simulink model "BEV_Laengsdynamikmodell_v2"  (R2023b)
settings: configuration reference "SharedConfig" (kept outside this file)
undefined symbols (not defined in the file): acc_cycle_flag, Analyse, battery, battery_builder_rtmsupport, config_battery, config_gearbox, config_Inverter, config_motor, config_vehicle, GB, gcbh, gearbox_map, k_FW, ModuleAssembly1, ModuleType1, motormap, motormap2
libraries: powerlib x37, nesl_utility x18, GD_Batterymodel_NSGAII_1_lib x12, BatteryProtection x9, fl_lib x7, dspstat3 x4, simulink x3, eePmsmCurrentReferenceGen x2, spsControlledCurrentSourceLib x2, spsVoltageMeasurementLib x2, batt_lib x1, BatteryBalancing x1
(part 3 of 6)

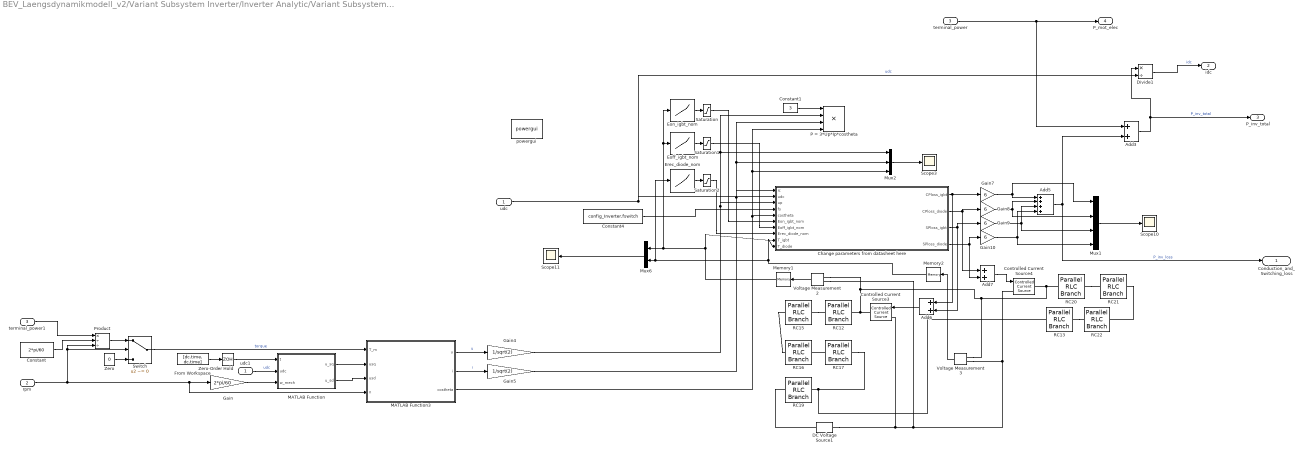
== system BEV_Laengsdynamikmodell_v2/Variant Subsystem Inverter/Inverter Analytic/Variant Subsystem/IM_Inverter_IGBT_Analytic ==
  udc : Inport
  rpm : Inport  Port=2
  terminal_power : Inport  Port=3
  Add3 : Sum
  Add5 : Sum  Inputs=++++
  Add6 : Sum
  Add7 : Sum
  Change parameters from datasheet here : MATLAB Function  TreatAsAtomicUnit=on
  Constant : Constant  Value=2*pi/60
  Constant1 : Constant  Value=3
  Constant4 : Constant  Value=config_Inverter.fswitch
  Controlled Current Source3 : powerlib/Electrical Sources/Controlled Current Source  Initialize=on  Source_Type=AC  Amplitude=0  Phase=0  Frequency=0  Measurements=None
  Controlled Current Source4 : powerlib/Electrical Sources/Controlled Current Source  Initialize=on  Source_Type=AC  Amplitude=0  Phase=0  Frequency=0  Measurements=None
  DC Voltage Source1 : powerlib/Electrical Sources/DC Voltage Source  Amplitude=25  Measurements=None
  Divide1 : Product  Inputs=*/
  Eoff_igbt_nom : Lookup_n-D  NumberOfTableDimensions=1  BreakpointsForDimension1=[25, 150, 175]  Table="[23.5*1e-3,  29*1e-3,  30*1e-3]"  InternalRulePriority=Speed  RndMeth=Simplest
  Eon_igbt_nom : Lookup_n-D  NumberOfTableDimensions=1  BreakpointsForDimension1=[25, 150, 175]  Table="[13.5*1e-3,  17.5*1e-3,  18*1e-3]"  InternalRulePriority=Speed  RndMeth=Simplest
  Erec_diode_nom : Lookup_n-D  NumberOfTableDimensions=1  BreakpointsForDimension1=[25, 150, 175]  Table="[7*1e-3,  13*1e-3,  15*1e-3]"  InternalRulePriority=Speed  RndMeth=Simplest
  From Workspace : FromWorkspace  VariableName=[dc.time, dc.time]
  Gain : Gain  Gain=2*pi/60
  Gain{7..10} (4 alike) : Gain  Gain=6
  Gain4 : Gain  Gain=1/sqrt(2)
  Gain5 : Gain  Gain=1/sqrt(2)
  MATLAB Function : MATLAB Function  TreatAsAtomicUnit=on
  MATLAB Function3 : MATLAB Function  TreatAsAtomicUnit=on
  Memory1 : Memory  InitialCondition=25  InheritSampleTime=on
  Memory2 : Memory  InitialCondition=25  InheritSampleTime=on
  Mux1 : Mux
  Mux2 : Mux  Inputs=3
  Mux6 : Mux  Inputs=2
  P = 3*Up*Ip*costheta : Product  Inputs=4
  Product : Product  Inputs=*//
  RC12 : powerlib/Elements/Parallel RLC Branch  LConnTagsString=a  RConnTagsString=__new0  BranchType=RC  Resistance=config_Inverter.R1igbt  Inductance=1e-3  SetiL0=off  InitialCurrent=0  Capacitance=config_Inverter.C1igbt  Setx0=off  InitialVoltage=0  Measurements=None
  RC13 : powerlib/Elements/Parallel RLC Branch  LConnTagsString=a  RConnTagsString=__new0  BranchType=RC  Resistance=config_Inverter.R4diode  Inductance=1e-3  SetiL0=off  InitialCurrent=0  Capacitance=config_Inverter.C4diode  Setx0=off  InitialVoltage=0  Measurements=None
  RC15 : powerlib/Elements/Parallel RLC Branch  LConnTagsString=a  RConnTagsString=__new0  BranchType=RC  Resistance=config_Inverter.R2igbt  Inductance=1e-3  SetiL0=off  InitialCurrent=0  Capacitance=config_Inverter.C2igbt  Setx0=off  InitialVoltage=0  Measurements=None
  RC16 : powerlib/Elements/Parallel RLC Branch  LConnTagsString=a  RConnTagsString=__new0  BranchType=RC  Resistance=config_Inverter.R3igbt  Inductance=1e-3  SetiL0=off  InitialCurrent=0  Capacitance=config_Inverter.C3igbt  Setx0=off  InitialVoltage=0  Measurements=None
  RC17 : powerlib/Elements/Parallel RLC Branch  LConnTagsString=a  RConnTagsString=__new0  BranchType=RC  Resistance=config_Inverter.R4igbt  Inductance=1e-3  SetiL0=off  InitialCurrent=0  Capacitance=config_Inverter.C4igbt  Setx0=off  InitialVoltage=0  Measurements=None
  RC19 : powerlib/Elements/Parallel RLC Branch  LConnTagsString=a  RConnTagsString=__new0  BranchType=R  Resistance=config_Inverter.R6igbt  Inductance=1e-3  SetiL0=off  InitialCurrent=0  Capacitance=175  Setx0=on  InitialVoltage=0  Measurements=None
  RC20 : powerlib/Elements/Parallel RLC Branch  LConnTagsString=a  RConnTagsString=__new0  BranchType=RC  Resistance=config_Inverter.R1diode  Inductance=1e-3  SetiL0=off  InitialCurrent=0  Capacitance=config_Inverter.C1diode  Setx0=off  InitialVoltage=0  Measurements=None
  RC21 : powerlib/Elements/Parallel RLC Branch  LConnTagsString=a  RConnTagsString=__new0  BranchType=RC  Resistance=config_Inverter.R2diode  Inductance=1e-3  SetiL0=off  InitialCurrent=0  Capacitance=config_Inverter.C2diode  Setx0=off  InitialVoltage=0  Measurements=None
  RC22 : powerlib/Elements/Parallel RLC Branch  LConnTagsString=a  RConnTagsString=__new0  BranchType=RC  Resistance=config_Inverter.R3diode  Inductance=1e-3  SetiL0=off  InitialCurrent=0  Capacitance=config_Inverter.C3diode  Setx0=off  InitialVoltage=0  Measurements=None
  Saturation : Saturate  UpperLimit=18*1e-3  LowerLimit=13.5*1e-3
  Saturation1 : Saturate  UpperLimit=30*1e-3  LowerLimit=23.5*1e-3
  Saturation2 : Saturate  UpperLimit=15*1e-3  LowerLimit=7*1e-3
  Scope10 : Scope
  Scope11 : Scope
  Scope3 : Scope
  Switch : Switch  Criteria=u2 ~= 0  SaturateOnIntegerOverflow=off  InputSameDT=off
  Voltage Measurement2 : powerlib/Measurements/Voltage Measurement  PhasorSimulation=off  OutputType=Complex  PSBequivalent=0
  Voltage Measurement3 : powerlib/Measurements/Voltage Measurement  PhasorSimulation=off  OutputType=Complex  PSBequivalent=0
  Zero : Constant  Value=0  OutDataTypeStr=Inherit: Inherit via back propagation
  Zero-Order Hold : ZeroOrderHold  SampleTime=-1
  powergui : powerlib/powergui  Priority=1  SimulationMode=Discrete  SampleTime=1  frequency=60  Iterations=50  frequencyindice=0  Pbase=100e6  ErrMax=1e-4  UnitsV=kV  UnitsW=MW  buscounter=0  FunctionMessages=on  echomessages=on  EnableUseOfTLC=off  CurrentSourceSwitches=off  DisableSnubberDevices=off  DisableRonSwitches=off  DisableVfSwitches=off  DisplayEquations=off  AutomaticDiscreteSolvers=off  SolverType=Backward Euler  Interpol=off  ExternalGateDelay=off  methode=off  Ts=100  x0status=blocks  SPID=off  SwTol=0  HookPort=off  NonlinearTolerance=1e-4  nMaxIteration=100  ContinueOnMaxIteration=off  RestoreLinks=warning  ResistiveCurrentMeasurement=off  Frange=[0:2:500]  Ylog=off  Xlog=on  ShowGrid=off  save=off  variable=ZData  structure=0  ZoomFFT=off  StartTime=0.0  cycles=1  DisplayStyle=1  fundamental=60  FreqAxis=off  MaxFrequency=1000  frequencyindicesteady=1  RmsSteady=1  display=off
  terminal_power1 : InportShadow  Port=3
  udc1 : InportShadow
  Conduction_and_Switching_loss : Outport
  idc : Outport  Port=2
  P_inv_total : Outport  Port=3
  P_mot_elec : Outport  Port=4
  wires:
  Eon_igbt_nom/1 -> Saturation/1
  Erec_diode_nom/1 -> Saturation2/1
  Eoff_igbt_nom/1 -> Saturation1/1
  Gain4/1 -> Change parameters from datasheet here/3(up), Mux2/1, P = 3*Up*Ip*costheta/2
  Saturation1/1 -> Change parameters from datasheet here/7(Eoff_igbt_nom)
  Switch/1 -> MATLAB Function3/1(T_m)  "torque"
  Divide1/1 -> idc/1  "idc"
  Voltage Measurement3/1 -> Memory2/1
  Change parameters from datasheet here/2(CPloss_diode) -> Add7/1, Gain8/1
  Add7/1 -> Controlled Current Source4/1
  Gain8/1 -> Add5/2, Mux1/2
  Change parameters from datasheet here/3(SPloss_igbt) -> Add6/2, Gain9/1
  Add3/1 -> Divide1/1, P_inv_total/1  "P_inv_total"
  Voltage Measurement2/1 -> Memory1/1
  Mux6/1 -> Scope11/1
  Saturation2/1 -> Change parameters from datasheet here/8(Erec_diode_nom)
  Saturation/1 -> Change parameters from datasheet here/6(Eon_igbt_nom)
  Change parameters from datasheet here/4(SPloss_diode) -> Add7/2, Gain10/1
  Gain9/1 -> Add5/3, Mux1/3
  Mux1/1 -> Scope10/1
  Gain7/1 -> Add5/1, Mux1/1
  Change parameters from datasheet here/1(CPloss_igbt) -> Gain7/1, Add6/1
  Constant4/1 -> Change parameters from datasheet here/4(fs)
  Memory1/1 -> Change parameters from datasheet here/9(T_igbt), Mux6/1, Eoff_igbt_nom/1, Eon_igbt_nom/1
  Memory2/1 -> Mux6/2, Erec_diode_nom/1, Change parameters from datasheet here/10(T_diode)
  Gain10/1 -> Mux1/4, Add5/4
  Constant1/1 -> P = 3*Up*Ip*costheta/1
  Add5/1 -> Add3/2, Conduction_and_Switching_loss/1  "P_inv_loss"
  Add6/1 -> Controlled Current Source3/1
  Mux2/1 -> Scope3/1
  udc/1 -> Divide1/2, Change parameters from datasheet here/2(udc)  "udc"
  MATLAB Function3/3(costheta) -> Mux2/3, P = 3*Up*Ip*costheta/4, Change parameters from datasheet here/5(costheta)
  Gain5/1 -> Change parameters from datasheet here/1(ic), Mux2/2, P = 3*Up*Ip*costheta/3
  MATLAB Function3/1(u) -> Gain4/1  "u"
  MATLAB Function3/2(i) -> Gain5/1  "i"
  MATLAB Function/1(u_sq) -> MATLAB Function3/2(usq)
  MATLAB Function/2(u_sd) -> MATLAB Function3/3(usd)
  Gain/1 -> MATLAB Function/3(w_mech)
  udc1/1 -> MATLAB Function/2(udc)  "udc"
  terminal_power/1 -> Add3/1, P_mot_elec/1
  Zero/1 -> Switch/3
  rpm/1 -> Switch/2, Product/3, MATLAB Function3/4(n), Gain/1
  Constant/1 -> Product/2
  Product/1 -> Switch/1
  terminal_power1/1 -> Product/1
  From Workspace/1 -> Zero-Order Hold/1
  Zero-Order Hold/1 -> MATLAB Function/1(t)
  connections:
  RC15/RConn1 -- RC12/LConn1
  RC17/LConn1 -- RC16/RConn1
  RC15/LConn1 -- RC16/LConn1
  RC20/LConn1 -- RC21/RConn1
  DC Voltage Source1/RConn1 -- RC19/LConn1
  RC13/LConn1 -- RC22/RConn1
  RC21/LConn1 -- RC22/LConn1
  RC17/RConn1 -- RC13/RConn1 -- RC19/RConn1
  Voltage Measurement2/LConn2 -- Voltage Measurement3/LConn2 -- Controlled Current Source4/LConn1 -- DC Voltage Source1/LConn1 -- Controlled Current Source3/LConn1
  RC12/RConn1 -- Controlled Current Source3/RConn1 -- Voltage Measurement2/LConn1 -- Voltage Measurement3/LConn1 -- RC20/RConn1 -- Controlled Current Source4/RConn1

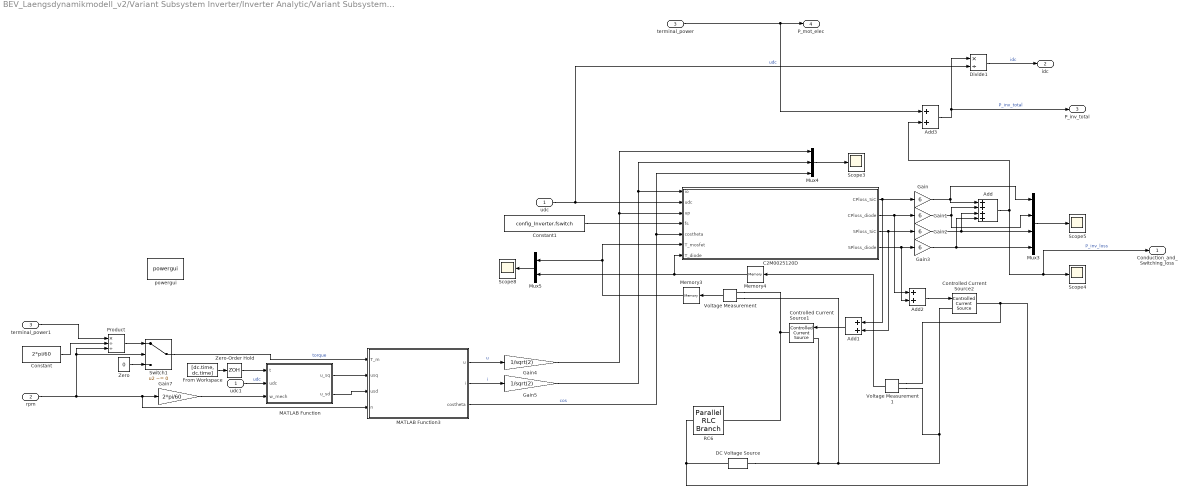
== system BEV_Laengsdynamikmodell_v2/Variant Subsystem Inverter/Inverter Analytic/Variant Subsystem/IM_Inverter_SiC-MOSFET_Analytic ==
  udc : Inport
  rpm : Inport  Port=2
  terminal_power : Inport  Port=3
  Add : Sum  Inputs=++++
  Add1 : Sum
  Add2 : Sum
  Add3 : Sum
  C2M0025120D : MATLAB Function  TreatAsAtomicUnit=on
  Constant : Constant  Value=2*pi/60
  Constant1 : Constant  Value=config_Inverter.fswitch
  Controlled Current Source1 : powerlib/Electrical Sources/Controlled Current Source  Initialize=on  Source_Type=AC  Amplitude=0  Phase=0  Frequency=0  Measurements=None
  Controlled Current Source2 : powerlib/Electrical Sources/Controlled Current Source  Initialize=on  Source_Type=AC  Amplitude=0  Phase=0  Frequency=0  Measurements=None
  DC Voltage Source : powerlib/Electrical Sources/DC Voltage Source  Amplitude=25  Measurements=None
  Divide1 : Product  Inputs=*/
  From Workspace : FromWorkspace  VariableName=[dc.time, dc.time]
  Gain{,1..3} (4 alike) : Gain  Gain=6
  Gain4 : Gain  Gain=1/sqrt(2)
  Gain5 : Gain  Gain=1/sqrt(2)
  Gain7 : Gain  Gain=2*pi/60
  MATLAB Function : MATLAB Function  TreatAsAtomicUnit=on
  MATLAB Function3 : MATLAB Function  TreatAsAtomicUnit=on
  Memory3 : Memory  InitialCondition=25  InheritSampleTime=on
  Memory4 : Memory  InitialCondition=25  InheritSampleTime=on
  Mux3 : Mux
  Mux4 : Mux  Inputs=3
  Mux5 : Mux  Inputs=2
  Product : Product  Inputs=*//
  RC6 : powerlib/Elements/Parallel RLC Branch  LConnTagsString=a  RConnTagsString=__new0  BranchType=R  Resistance=config_Inverter.Rmosfet  Inductance=1e-3  SetiL0=off  InitialCurrent=0  Capacitance=175  Setx0=on  InitialVoltage=0  Measurements=None
  Scope{3..5,8} (4 alike) : Scope
  Switch1 : Switch  Criteria=u2 ~= 0  SaturateOnIntegerOverflow=off  InputSameDT=off
  Voltage Measurement : powerlib/Measurements/Voltage Measurement  PhasorSimulation=off  OutputType=Complex  PSBequivalent=0
  Voltage Measurement1 : powerlib/Measurements/Voltage Measurement  PhasorSimulation=off  OutputType=Complex  PSBequivalent=0
  Zero : Constant  Value=0  OutDataTypeStr=Inherit: Inherit via back propagation
  Zero-Order Hold : ZeroOrderHold  SampleTime=-1
  powergui : powerlib/powergui  Priority=1  SimulationMode=Discrete  SampleTime=1  frequency=60  Iterations=50  frequencyindice=0  Pbase=100e6  ErrMax=1e-4  UnitsV=kV  UnitsW=MW  buscounter=0  FunctionMessages=on  echomessages=on  EnableUseOfTLC=off  CurrentSourceSwitches=off  DisableSnubberDevices=off  DisableRonSwitches=off  DisableVfSwitches=off  DisplayEquations=off  AutomaticDiscreteSolvers=off  SolverType=Backward Euler  Interpol=off  ExternalGateDelay=off  methode=off  Ts=100  x0status=blocks  SPID=off  SwTol=0  HookPort=off  NonlinearTolerance=1e-4  nMaxIteration=100  ContinueOnMaxIteration=off  RestoreLinks=warning  ResistiveCurrentMeasurement=off  Frange=[0:2:500]  Ylog=off  Xlog=on  ShowGrid=off  save=off  variable=ZData  structure=0  ZoomFFT=off  StartTime=0.0  cycles=1  DisplayStyle=1  fundamental=60  FreqAxis=off  MaxFrequency=1000  frequencyindicesteady=1  RmsSteady=1  display=off
  terminal_power1 : InportShadow  Port=3
  udc1 : InportShadow
  Conduction_and_Switching_loss : Outport
  idc : Outport  Port=2
  P_inv_total : Outport  Port=3
  P_mot_elec : Outport  Port=4
  wires:
  terminal_power/1 -> Add3/1, P_mot_elec/1
  Add3/1 -> Divide1/1, P_inv_total/1  "P_inv_total"
  Gain5/1 -> Mux4/2, C2M0025120D/1(io)
  Gain4/1 -> Mux4/1, C2M0025120D/3(up)
  udc/1 -> C2M0025120D/2(udc), Divide1/2  "udc"
  Divide1/1 -> idc/1  "idc"
  Add/1 -> Scope4/1, Conduction_and_Switching_loss/1, Add3/2  "P_inv_loss"
  MATLAB Function3/3(costheta) -> Mux4/3, C2M0025120D/5(costheta)  "cos"
  MATLAB Function3/2(i) -> Gain5/1  "i"
  Mux3/1 -> Scope5/1
  Mux4/1 -> Scope3/1
  Voltage Measurement/1 -> Memory3/1
  Mux5/1 -> Scope8/1
  C2M0025120D/2(CPloss_diode) -> Gain1/1, Add2/1
  Constant1/1 -> C2M0025120D/4(fs)
  C2M0025120D/3(SPloss_SiC) -> Gain2/1, Add1/2
  Voltage Measurement1/1 -> Memory4/1
  Add2/1 -> Controlled Current Source2/1
  Memory4/1 -> Mux5/2, C2M0025120D/7(T_diode)
  Add1/1 -> Controlled Current Source1/1
  Gain/1 -> Add/1, Mux3/1
  C2M0025120D/4(SPloss_diode) -> Gain3/1, Add2/2
  Gain1/1 -> Add/2, Mux3/2
  Gain2/1 -> Add/3, Mux3/3
  C2M0025120D/1(CPloss_SiC) -> Gain/1, Add1/1
  Memory3/1 -> C2M0025120D/6(T_mosfet), Mux5/1
  Gain3/1 -> Mux3/4, Add/4
  MATLAB Function/1(u_sq) -> MATLAB Function3/2(usq)
  MATLAB Function/2(u_sd) -> MATLAB Function3/3(usd)
  MATLAB Function3/1(u) -> Gain4/1  "u"
  terminal_power1/1 -> Product/1
  udc1/1 -> MATLAB Function/2(udc)  "udc"
  rpm/1 -> Switch1/2, Product/3, MATLAB Function3/4(n), Gain7/1
  Gain7/1 -> MATLAB Function/3(w_mech)
  Zero/1 -> Switch1/3
  Product/1 -> Switch1/1
  Constant/1 -> Product/2
  Switch1/1 -> MATLAB Function3/1(T_m)  "torque"
  From Workspace/1 -> Zero-Order Hold/1
  Zero-Order Hold/1 -> MATLAB Function/1(t)
  connections:
  RC6/RConn1 -- Controlled Current Source1/RConn1 -- Voltage Measurement/LConn1
  Controlled Current Source2/LConn1 -- Voltage Measurement/LConn2 -- Controlled Current Source1/LConn1 -- DC Voltage Source/LConn1 -- Voltage Measurement1/LConn2
  Voltage Measurement1/LConn1 -- Controlled Current Source2/RConn1 -- RC6/LConn1 -- DC Voltage Source/RConn1

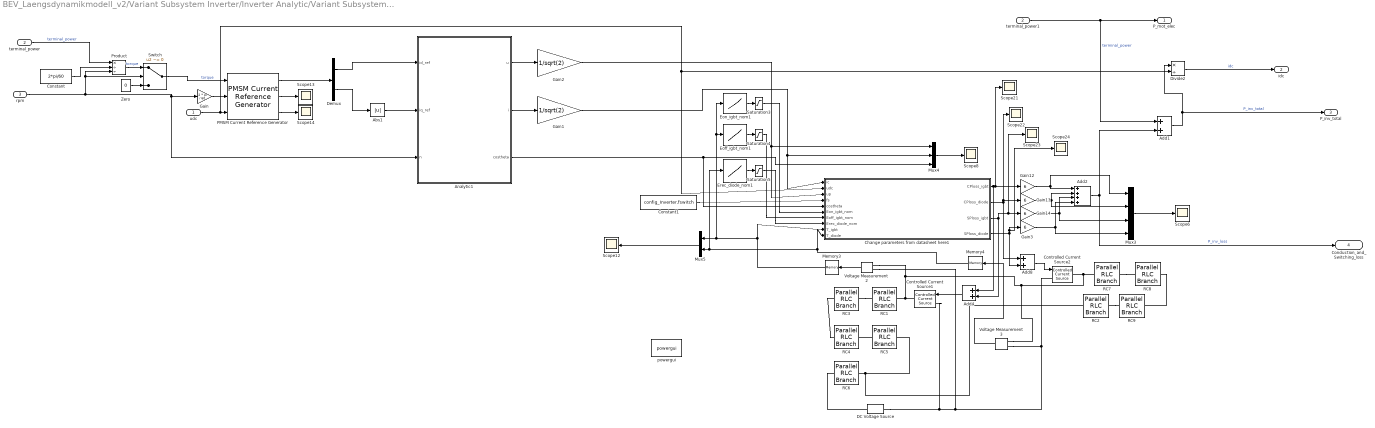
== system BEV_Laengsdynamikmodell_v2/Variant Subsystem Inverter/Inverter Analytic/Variant Subsystem/PMSM_Inverter_IBGT_Analytic ==
  udc : Inport
  terminal_power : Inport  Port=2
  rpm : Inport  Port=3
  Abs1 : Abs  SaturateOnIntegerOverflow=off
  Add1 : Sum
  Add2 : Sum  Inputs=++++
  Add4 : Sum
  Add8 : Sum
  Analytic1 : MATLAB Function  TreatAsAtomicUnit=on
  Change parameters from datasheet here1 : MATLAB Function  TreatAsAtomicUnit=on
  Constant : Constant  Value=2*pi/60
  Constant1 : Constant  Value=config_Inverter.fswitch
  Controlled Current Source1 : powerlib/Electrical Sources/Controlled Current Source  Initialize=on  Source_Type=AC  Amplitude=0  Phase=0  Frequency=0  Measurements=None
  Controlled Current Source2 : powerlib/Electrical Sources/Controlled Current Source  Initialize=on  Source_Type=AC  Amplitude=0  Phase=0  Frequency=0  Measurements=None
  DC Voltage Source : powerlib/Electrical Sources/DC Voltage Source  Amplitude=25  Measurements=None
  Demux : Demux  Outputs=2
  Divide2 : Product  Inputs=*/
  Eoff_igbt_nom1 : Lookup_n-D  NumberOfTableDimensions=1  BreakpointsForDimension1=[25, 150, 175]  Table="[23.5*1e-3,  29*1e-3,  30*1e-3]"  InternalRulePriority=Speed  RndMeth=Simplest
  Eon_igbt_nom1 : Lookup_n-D  NumberOfTableDimensions=1  BreakpointsForDimension1=[25, 150, 175]  Table="[13.5*1e-3,  17.5*1e-3,  18*1e-3]"  InternalRulePriority=Speed  RndMeth=Simplest
  Erec_diode_nom1 : Lookup_n-D  NumberOfTableDimensions=1  BreakpointsForDimension1=[25, 150, 175]  Table="[7*1e-3,  13*1e-3,  15*1e-3]"  InternalRulePriority=Speed  RndMeth=Simplest
  Gain : Gain  Gain=2 * pi / 60
  Gain1 : Gain  Gain=1/sqrt(2)
  Gain{3,12..14} (4 alike) : Gain  Gain=6
  Gain2 : Gain  Gain=1/sqrt(2)
  Memory3 : Memory  InitialCondition=25  InheritSampleTime=on
  Memory4 : Memory  InitialCondition=25  InheritSampleTime=on
  Mux3 : Mux
  Mux4 : Mux  Inputs=3
  Mux5 : Mux  Inputs=2
  PMSM Current Reference Generator : eePmsmCurrentReferenceGen/PMSM Current Reference Generator  Vnom=360  Pmax=150000  Tmax=350  Ts=-1  RefType=Automatically generated lookup-table  rpmVec=[0, 3000]  TqVec=[-100, 0, 100]  VdcVec=[300, 350]  PWMMode=SPWM: sinusoidal PWM  ModFactor=0.97  idMatrix=zeros(2,3,2)  iqMatrix=zeros(2,3,2)  p=6  psim=0.0347  Ld=0.0000436  Lq=0.0000975  Rs=0.0049  RefExpEnable=0
  Product : Product  Inputs=*//
  RC1 : powerlib/Elements/Parallel RLC Branch  LConnTagsString=a  RConnTagsString=__new0  BranchType=RC  Resistance=config_Inverter.R1igbt  Inductance=1e-3  SetiL0=off  InitialCurrent=0  Capacitance=config_Inverter.C1igbt  Setx0=off  InitialVoltage=0  Measurements=None
  RC2 : powerlib/Elements/Parallel RLC Branch  LConnTagsString=a  RConnTagsString=__new0  BranchType=RC  Resistance=config_Inverter.R4diode  Inductance=1e-3  SetiL0=off  InitialCurrent=0  Capacitance=config_Inverter.C4diode  Setx0=off  InitialVoltage=0  Measurements=None
  RC3 : powerlib/Elements/Parallel RLC Branch  LConnTagsString=a  RConnTagsString=__new0  BranchType=RC  Resistance=config_Inverter.R2igbt  Inductance=1e-3  SetiL0=off  InitialCurrent=0  Capacitance=config_Inverter.C2igbt  Setx0=off  InitialVoltage=0  Measurements=None
  RC4 : powerlib/Elements/Parallel RLC Branch  LConnTagsString=a  RConnTagsString=__new0  BranchType=RC  Resistance=config_Inverter.R3igbt  Inductance=1e-3  SetiL0=off  InitialCurrent=0  Capacitance=config_Inverter.C3igbt  Setx0=off  InitialVoltage=0  Measurements=None
  RC5 : powerlib/Elements/Parallel RLC Branch  LConnTagsString=a  RConnTagsString=__new0  BranchType=RC  Resistance=config_Inverter.R4igbt  Inductance=1e-3  SetiL0=off  InitialCurrent=0  Capacitance=config_Inverter.C4igbt  Setx0=off  InitialVoltage=0  Measurements=None
  RC6 : powerlib/Elements/Parallel RLC Branch  LConnTagsString=a  RConnTagsString=__new0  BranchType=R  Resistance=config_Inverter.R6igbt  Inductance=1e-3  SetiL0=off  InitialCurrent=0  Capacitance=175  Setx0=on  InitialVoltage=0  Measurements=None
  RC7 : powerlib/Elements/Parallel RLC Branch  LConnTagsString=a  RConnTagsString=__new0  BranchType=RC  Resistance=config_Inverter.R1diode  Inductance=1e-3  SetiL0=off  InitialCurrent=0  Capacitance=config_Inverter.C1diode  Setx0=off  InitialVoltage=0  Measurements=None
  RC8 : powerlib/Elements/Parallel RLC Branch  LConnTagsString=a  RConnTagsString=__new0  BranchType=RC  Resistance=config_Inverter.R2diode  Inductance=1e-3  SetiL0=off  InitialCurrent=0  Capacitance=config_Inverter.C2diode  Setx0=off  InitialVoltage=0  Measurements=None
  RC9 : powerlib/Elements/Parallel RLC Branch  LConnTagsString=a  RConnTagsString=__new0  BranchType=RC  Resistance=config_Inverter.R3diode  Inductance=1e-3  SetiL0=off  InitialCurrent=0  Capacitance=config_Inverter.C3diode  Setx0=off  InitialVoltage=0  Measurements=None
  Saturation3 : Saturate  UpperLimit=18*1e-3  LowerLimit=13.5*1e-3
  Saturation4 : Saturate  UpperLimit=30*1e-3  LowerLimit=23.5*1e-3
  Saturation5 : Saturate  UpperLimit=15*1e-3  LowerLimit=7*1e-3
  Scope{6,8,12..14,21..24} (9 alike) : Scope
  Switch : Switch  Criteria=u2 ~= 0  SaturateOnIntegerOverflow=off  InputSameDT=off
  Voltage Measurement2 : powerlib/Measurements/Voltage Measurement  PhasorSimulation=off  OutputType=Complex  PSBequivalent=0
  Voltage Measurement3 : powerlib/Measurements/Voltage Measurement  PhasorSimulation=off  OutputType=Complex  PSBequivalent=0
  Zero : Constant  Value=0  OutDataTypeStr=Inherit: Inherit via back propagation
  powergui : powerlib/powergui  Priority=1  SimulationMode=Discrete  SampleTime=1  frequency=60  Iterations=50  frequencyindice=0  Pbase=100e6  ErrMax=1e-4  UnitsV=kV  UnitsW=MW  buscounter=0  FunctionMessages=on  echomessages=on  EnableUseOfTLC=off  CurrentSourceSwitches=off  DisableSnubberDevices=off  DisableRonSwitches=off  DisableVfSwitches=off  DisplayEquations=off  AutomaticDiscreteSolvers=off  SolverType=Backward Euler  Interpol=off  ExternalGateDelay=off  methode=off  Ts=100  x0status=blocks  SPID=off  SwTol=0  HookPort=off  NonlinearTolerance=1e-4  nMaxIteration=100  ContinueOnMaxIteration=off  RestoreLinks=warning  ResistiveCurrentMeasurement=off  Frange=[0:2:500]  Ylog=off  Xlog=on  ShowGrid=off  save=off  variable=ZData  structure=0  ZoomFFT=off  StartTime=0.0  cycles=1  DisplayStyle=1  fundamental=60  FreqAxis=off  MaxFrequency=1000  frequencyindicesteady=1  RmsSteady=1  display=off
  terminal_power1 : InportShadow  Port=2
  P_mot_elec : Outport
  idc : Outport  Port=2
  P_inv_total : Outport  Port=3
  Conduction_and_Switching_loss : Outport  Port=4
  wires:
  PMSM Current Reference Generator/2 -> Scope13/1
  Eon_igbt_nom1/1 -> Saturation3/1
  Divide2/1 -> idc/1  "idc"
  Voltage Measurement2/1 -> Memory3/1
  Add8/1 -> Controlled Current Source2/1
  Change parameters from datasheet here1/3(SPloss_igbt) -> Scope23/1, Gain14/1, Add4/2
  Change parameters from datasheet here1/1(CPloss_igbt) -> Add4/1, Gain12/1, Scope21/1
  Gain2/1 -> Change parameters from datasheet here1/3(up), Mux4/1
  Add4/1 -> Controlled Current Source1/1
  Constant1/1 -> Change parameters from datasheet here1/4(fs)
  Eoff_igbt_nom1/1 -> Saturation4/1
  Saturation4/1 -> Change parameters from datasheet here1/7(Eoff_igbt_nom)
  PMSM Current Reference Generator/3 -> Scope14/1
  Demux/2 -> Abs1/1
  Change parameters from datasheet here1/2(CPloss_diode) -> Scope22/1, Gain13/1, Add8/1
  Voltage Measurement3/1 -> Memory4/1
  Memory3/1 -> Change parameters from datasheet here1/9(T_igbt), Eoff_igbt_nom1/1, Eon_igbt_nom1/1, Mux5/1
  Mux4/1 -> Scope8/1
  Mux5/1 -> Scope12/1
  Demux/1 -> Analytic1/1(id_ref)
  Memory4/1 -> Erec_diode_nom1/1, Mux5/2, Change parameters from datasheet here1/10(T_diode)
  Saturation5/1 -> Change parameters from datasheet here1/8(Erec_diode_nom)
  Add1/1 -> Divide2/1, P_inv_total/1  "P_inv_total"
  Analytic1/1(u) -> Gain2/1
  Erec_diode_nom1/1 -> Saturation5/1
  Mux3/1 -> Scope6/1
  Gain14/1 -> Mux3/3, Add2/3
  Gain/1 -> PMSM Current Reference Generator/2
  Add2/1 -> Conduction_and_Switching_loss/1, Add1/2  "P_inv_loss"
  Change parameters from datasheet here1/4(SPloss_diode) -> Scope24/1, Gain3/1, Add8/2
  Analytic1/2(i) -> Gain1/1
  PMSM Current Reference Generator/1 -> Demux/1
  Saturation3/1 -> Change parameters from datasheet here1/6(Eon_igbt_nom)
  Abs1/1 -> Analytic1/2(iq_ref)
  Gain13/1 -> Mux3/2, Add2/2
  rpm/1 -> Switch/2, Product/3, Analytic1/3(n), Gain/1
  terminal_power1/1 -> P_mot_elec/1, Add1/1  "terminal_power"
  Gain1/1 -> Change parameters from datasheet here1/1(ic), Mux4/2
  Gain12/1 -> Mux3/1, Add2/1
  udc/1 -> PMSM Current Reference Generator/3, Change parameters from datasheet here1/2(udc), Divide2/2
  Switch/1 -> PMSM Current Reference Generator/1  "torque"
  Gain3/1 -> Add2/4, Mux3/4
  Analytic1/3(costheta) -> Mux4/3, Change parameters from datasheet here1/5(costheta)
  terminal_power/1 -> Product/1  "terminal_power"
  Constant/1 -> Product/2
  Product/1 -> Switch/1  "torque"
  Zero/1 -> Switch/3
  connections:
  RC3/RConn1 -- RC1/LConn1
  RC7/LConn1 -- RC8/RConn1
  DC Voltage Source/RConn1 -- RC6/LConn1
  RC3/LConn1 -- RC4/LConn1
  RC5/LConn1 -- RC4/RConn1
  RC8/LConn1 -- RC9/LConn1
  Controlled Current Source1/LConn1 -- DC Voltage Source/LConn1 -- Voltage Measurement2/LConn1 -- Voltage Measurement3/LConn1 -- Controlled Current Source2/LConn1
  RC2/LConn1 -- RC9/RConn1
  RC5/RConn1 -- RC6/RConn1 -- RC2/RConn1
  Controlled Current Source2/RConn1 -- RC7/RConn1 -- Voltage Measurement3/LConn2 -- Voltage Measurement2/LConn2 -- Controlled Current Source1/RConn1 -- RC1/RConn1

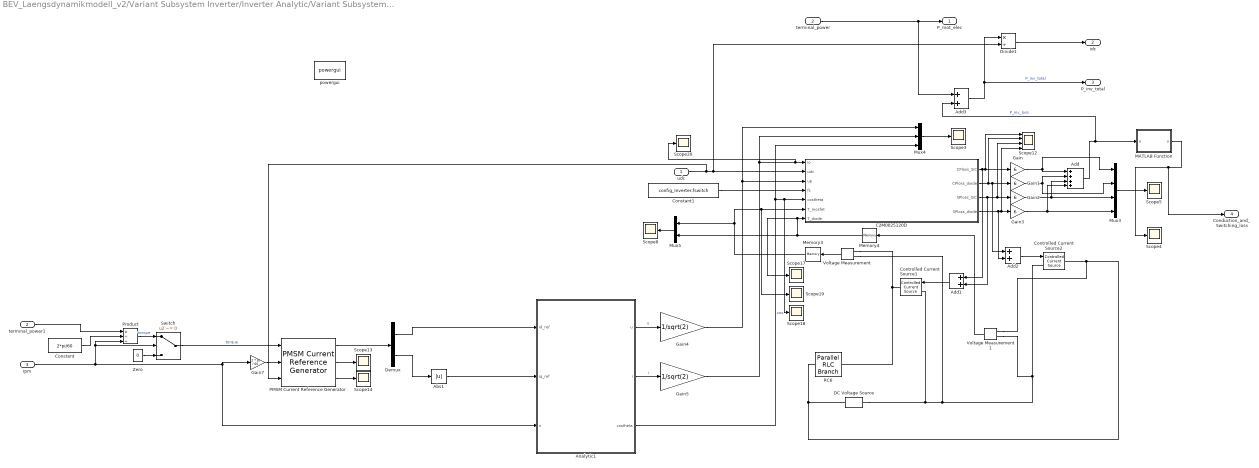
== system BEV_Laengsdynamikmodell_v2/Variant Subsystem Inverter/Inverter Analytic/Variant Subsystem/PMSM_Inverter_SiC-MOSFET_Analytic ==
  udc : Inport
  terminal_power : Inport  Port=2
  rpm : Inport  Port=3
  Abs1 : Abs  SaturateOnIntegerOverflow=off
  Add : Sum  Inputs=++++
  Add1 : Sum
  Add2 : Sum
  Add3 : Sum
  Analytic1 : MATLAB Function  TreatAsAtomicUnit=on
  C2M0025120D : MATLAB Function  TreatAsAtomicUnit=on
  Constant : Constant  Value=2*pi/60
  Constant1 : Constant  Value=config_Inverter.fswitch
  Controlled Current Source1 : spsControlledCurrentSourceLib/Controlled Current Source  Initialize=on  Source_Type=AC  Amplitude=0  Phase=0  Frequency=0  Measurements=None
  Controlled Current Source2 : spsControlledCurrentSourceLib/Controlled Current Source  Initialize=on  Source_Type=AC  Amplitude=0  Phase=0  Frequency=0  Measurements=None
  DC Voltage Source : spsDCVoltageSourceLib/DC Voltage Source  Amplitude=25  Measurements=None
  Demux : Demux  Outputs=2
  Divide1 : Product  Inputs=*/
  Gain{,1..3} (4 alike) : Gain  Gain=6
  Gain4 : Gain  Gain=1/sqrt(2)
  Gain5 : Gain  Gain=1/sqrt(2)
  Gain7 : Gain  Gain=2 * pi / 60
  MATLAB Function : MATLAB Function  TreatAsAtomicUnit=on
  Memory3 : Memory  InitialCondition=25  InheritSampleTime=on
  Memory4 : Memory  InitialCondition=25  InheritSampleTime=on
  Mux3 : Mux
  Mux4 : Mux  Inputs=3
  Mux5 : Mux  Inputs=2
  PMSM Current Reference Generator : eePmsmCurrentReferenceGen/PMSM Current Reference Generator  Vnom=360  Pmax=150000  Tmax=350  Ts=-1  RefType=Automatically generated lookup-table  rpmVec=[0, 3000]  TqVec=[-100, 0, 100]  VdcVec=[300, 350]  PWMMode=SPWM: sinusoidal PWM  ModFactor=0.97  idMatrix=zeros(2,3,2)  iqMatrix=zeros(2,3,2)  p=6  psim=0.0347  Ld=0.0000436  Lq=0.0000975  Rs=0.0049  RefExpEnable=0
  Product : Product  Inputs=*//
  RC6 : spsParallelRLCBranchLib/Parallel RLC Branch  LConnTagsString=a  RConnTagsString=__new0  BranchType=R  Resistance=config_Inverter.Rmosfet  Inductance=1e-3  SetiL0=off  InitialCurrent=0  Capacitance=175  Setx0=on  InitialVoltage=0  Measurements=None
  Scope12 : Scope  NumInputPorts=4
  Scope{3..5,8,13..14,17..20} (10 alike) : Scope
  Switch : Switch  Criteria=u2 ~= 0  SaturateOnIntegerOverflow=off  InputSameDT=off
  Voltage Measurement : spsVoltageMeasurementLib/Voltage Measurement  PhasorSimulation=off  OutputType=Complex  PSBequivalent=0
  Voltage Measurement1 : spsVoltageMeasurementLib/Voltage Measurement  PhasorSimulation=off  OutputType=Complex  PSBequivalent=0
  Zero : Constant  Value=0  OutDataTypeStr=Inherit: Inherit via back propagation
  powergui : spspowerguiLib/powergui  Priority=1  SimulationMode=Discrete  SampleTime=1  frequency=60  Iterations=50  frequencyindice=0  Pbase=100e6  ErrMax=1e-4  UnitsV=kV  UnitsW=MW  buscounter=0  FunctionMessages=on  echomessages=on  EnableUseOfTLC=off  CurrentSourceSwitches=off  DisableSnubberDevices=off  DisableRonSwitches=off  DisableVfSwitches=off  DisplayEquations=off  AutomaticDiscreteSolvers=off  SolverType=Backward Euler  Interpol=off  ExternalGateDelay=off  methode=off  Ts=100  x0status=blocks  SPID=off  SwTol=0  HookPort=off  NonlinearTolerance=1e-4  nMaxIteration=100  ContinueOnMaxIteration=off  RestoreLinks=warning  ResistiveCurrentMeasurement=off  Frange=[0:2:500]  Ylog=off  Xlog=on  ShowGrid=off  save=off  variable=ZData  structure=0  ZoomFFT=off  StartTime=0.0  cycles=1  DisplayStyle=1  fundamental=60  FreqAxis=off  MaxFrequency=1000  frequencyindicesteady=1  RmsSteady=1  display=off
  terminal_power1 : InportShadow  Port=2
  P_mot_elec : Outport
  idc : Outport  Port=2
  P_inv_total : Outport  Port=3
  Conduction_and_Switching_loss : Outport  Port=4
  wires:
  udc/1 -> PMSM Current Reference Generator/3, Divide1/2, C2M0025120D/2(udc)
  Gain1/1 -> Mux3/2, Add/2
  Gain4/1 -> Mux4/1, C2M0025120D/3(up)
  Memory3/1 -> Mux5/1, Scope19/1, C2M0025120D/6(T_mosfet)
  Add2/1 -> Controlled Current Source2/1
  Constant1/1 -> C2M0025120D/4(fs)
  Divide1/1 -> idc/1
  C2M0025120D/3(SPloss_SiC) -> Add1/2, Scope12/3, Gain2/1
  Analytic1/3(costheta) -> Mux4/3, Scope18/1, C2M0025120D/5(costheta)  "cos"
  Gain/1 -> Mux3/1, Add/1
  C2M0025120D/2(CPloss_diode) -> Scope12/2, Add2/1, Gain1/1
  Mux4/1 -> Scope3/1
  Gain5/1 -> Mux4/2, Scope20/1, C2M0025120D/1(io)
  terminal_power/1 -> P_mot_elec/1, Add3/1
  Memory4/1 -> Scope17/1, C2M0025120D/7(T_diode), Mux5/2
  Add/1 -> Add3/2, MATLAB Function/1(u)  "P_inv_loss"
  C2M0025120D/4(SPloss_diode) -> Scope12/4, Gain3/1, Add2/2
  Gain2/1 -> Mux3/3, Add/3
  Add1/1 -> Controlled Current Source1/1
  C2M0025120D/1(CPloss_SiC) -> Add1/1, Scope12/1, Gain/1
  Analytic1/2(i) -> Gain5/1  "i"
  Gain3/1 -> Add/4, Mux3/4
  Voltage Measurement1/1 -> Memory4/1
  Add3/1 -> P_inv_total/1, Divide1/1  "P_inv_total"
  Voltage Measurement/1 -> Memory3/1
  Mux5/1 -> Scope8/1
  Mux3/1 -> Scope5/1
  Analytic1/1(u) -> Gain4/1  "u"
  PMSM Current Reference Generator/3 -> Scope14/1
  PMSM Current Reference Generator/2 -> Scope13/1
  Switch/1 -> PMSM Current Reference Generator/1  "torque"
  Demux/2 -> Abs1/1
  rpm/1 -> Gain7/1, Analytic1/3(n), Switch/2, Product/3
  Gain7/1 -> PMSM Current Reference Generator/2
  Demux/1 -> Analytic1/1(id_ref)
  Abs1/1 -> Analytic1/2(iq_ref)
  PMSM Current Reference Generator/1 -> Demux/1
  Zero/1 -> Switch/3
  Constant/1 -> Product/2
  Product/1 -> Switch/1  "torque"
  terminal_power1/1 -> Product/1
  MATLAB Function/1(y) -> Conduction_and_Switching_loss/1, Scope4/1
  connections:
  Voltage Measurement/LConn1 -- Controlled Current Source1/RConn1 -- RC6/RConn1
  DC Voltage Source/RConn1 -- Controlled Current Source2/RConn1 -- Voltage Measurement1/LConn1 -- RC6/LConn1
  Voltage Measurement1/LConn2 -- DC Voltage Source/LConn1 -- Controlled Current Source1/LConn1 -- Voltage Measurement/LConn2 -- Controlled Current Source2/LConn1
